simulink model "PMSM_simplified"  (R2023a)
settings: Solver=VariableStepAuto  StartTime=0.0  StopTime=1  RelTol=1e-3
libraries: spsVoltageMeasurementLib x3, spsGroundLib x1, spsPermanentMagnetSynchronousMachineLib x1, spsThreePhaseProgrammableVoltageSourceLib x1, sps_lib x1
settings Model: Creator=siddh  LastModifiedBy=siddh

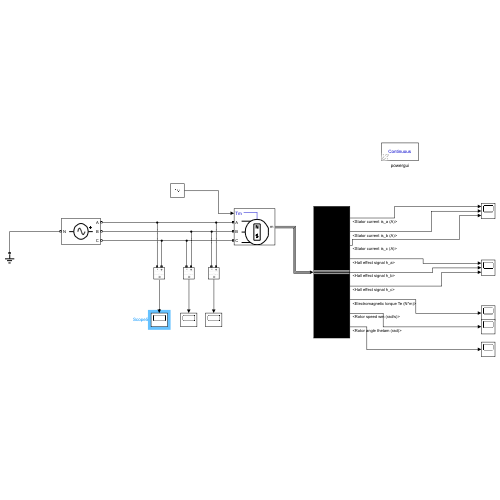
[thumbnail: Simulink's stored preview of the top-level diagram]
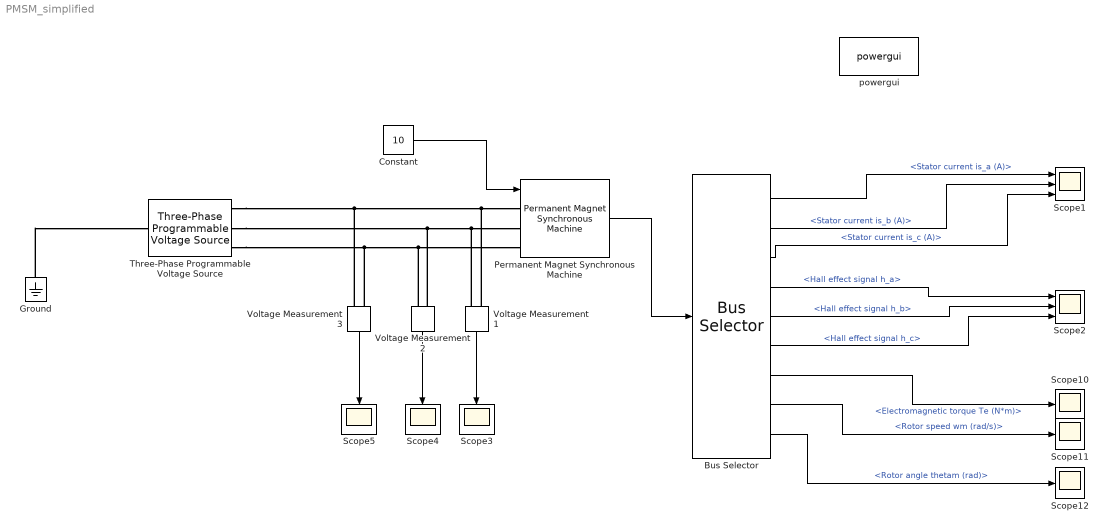
== system PMSM_simplified ==
  Bus Selector : BusSelector  OutputSignals=Stator current is_a (A),Stator current is_b (A),Stator current is_c (A),Hall effect signal h_a,Hall effect signal h_b,Hall effect signal h_c,Electromagnetic torque Te (N*m),Rotor speed wm (rad/s),Rotor angle thetam (rad)
  Constant : Constant  Value=10
  Ground : spsGroundLib/Ground  LConnTagsString=a
  Permanent Magnet Synchronous Machine : spsPermanentMagnetSynchronousMachineLib/Permanent Magnet Synchronous Machine  NbPhases=3  FluxDistribution=Sinusoidal  RotorType=Round  MechanicalLoad=Torque Tm  PresetModel=No  ShowDetailedParameters=on  MeasurementBus=off  Resistance=18.7  Inductance=8.5e-3  dqInductances=[8.5e-3,8.5e-3]  La=0.02682  MachineConstant=Flux linkage established by magnets (V.s)  Flux=0.1716  VoltageCst=62.2496  TorqueCst=0.5148  Flat=120  Mechanical=[2.26e-05 1.349e-05 2 0]  PolePairs=2  InitialConditions=[0,0, 0,0]  InitialConditions5ph=[0 0 0 0 0 0]  RefAngle=90 degrees behind phase A axis (modified Park)  IterativeDiscreteModel=Trapezoidal non iterative  TsBlock=-1  TsPowergui=0
  Scope1 : Scope  NumInputPorts=3
  Scope{3..5,10..12} (6 alike) : Scope
  Scope2 : Scope  NumInputPorts=3
  Three-Phase Programmable Voltage Source : spsThreePhaseProgrammableVoltageSourceLib/Three-Phase Programmable Voltage Source  PositiveSequence="[100  0 50]"  VariationEntity=None  VariationType=Table of time-amplitude pairs  VariationTypeAlt=Step  VariationStep=0.5  VariationRate=10  VariationMagnitude=0.3  VariationFrequency=2  VariationTiming=[1 2]  VariationPhaseA=off  Amplitudes=[1 0.8 1.2 1.0]  TimeValues=[0 0.1 0.15 0.2]  HarmonicGeneration=off  HarmonicA=[3 0.2 -25 0]  HarmonicB=[2 0.15 35 2]  Timing="[0.05  3]"  BusType=swing  Pref=0  Qref=0  Qmin=-inf  Qmax=inf
  Voltage Measurement1 : spsVoltageMeasurementLib/Voltage Measurement  PhasorSimulation=off  OutputType=Complex  PSBequivalent=0
  Voltage Measurement2 : spsVoltageMeasurementLib/Voltage Measurement  PhasorSimulation=off  OutputType=Complex  PSBequivalent=0
  Voltage Measurement3 : spsVoltageMeasurementLib/Voltage Measurement  PhasorSimulation=off  OutputType=Complex  PSBequivalent=0
  powergui : sps_lib/powergui  Priority=1  SimulationMode=Continuous  SampleTime=50e-6  frequency=60  Iterations=50  frequencyindice=0  Pbase=100e6  ErrMax=1e-4  UnitsV=kV  UnitsW=MW  buscounter=0  FunctionMessages=off  echomessages=off  EnableUseOfTLC=off  CurrentSourceSwitches=off  DisableSnubberDevices=off  DisableRonSwitches=off  DisableVfSwitches=off  DisplayEquations=off  AutomaticDiscreteSolvers=off  SolverType=Tustin/Backward Euler (TBE)  Interpol=off  ExternalGateDelay=off  methode=off  Ts=100  x0status=blocks  SPID=on  SwTol=0  HookPort=off  NonlinearTolerance=1e-4  nMaxIteration=100  ContinueOnMaxIteration=off  RestoreLinks=warning  ResistiveCurrentMeasurement=off  Frange=[0:2:500]  Ylog=off  Xlog=on  ShowGrid=off  save=off  variable=ZData  structure=0  ZoomFFT=off  StartTime=0.0  cycles=1  DisplayStyle=1  fundamental=60  FreqAxis=off  MaxFrequency=1000  frequencyindicesteady=1  RmsSteady=1  display=off
  wires:
  Bus Selector/6 -> Scope2/3  "<Hall effect signal h_c>"
  Bus Selector/7 -> Scope10/1  "<Electromagnetic torque Te (N*m)>"
  Constant/1 -> Permanent Magnet Synchronous Machine/1
  Permanent Magnet Synchronous Machine/1 -> Bus Selector/1
  Bus Selector/2 -> Scope1/2  "<Stator current is_b (A)>"
  Bus Selector/8 -> Scope11/1  "<Rotor speed wm (rad/s)>"
  Bus Selector/1 -> Scope1/1  "<Stator current is_a (A)>"
  Bus Selector/3 -> Scope1/3  "<Stator current is_c (A)>"
  Bus Selector/9 -> Scope12/1  "<Rotor angle thetam (rad)>"
  Bus Selector/4 -> Scope2/1  "<Hall effect signal h_a>"
  Bus Selector/5 -> Scope2/2  "<Hall effect signal h_b>"
  Voltage Measurement1/1 -> Scope3/1
  Voltage Measurement2/1 -> Scope4/1
  Voltage Measurement3/1 -> Scope5/1
  connections:
  Three-Phase Programmable Voltage Source/RConn1 -- Voltage Measurement3/LConn2 -- Voltage Measurement1/LConn1 -- Permanent Magnet Synchronous Machine/LConn1
  Three-Phase Programmable Voltage Source/RConn2 -- Voltage Measurement1/LConn2 -- Permanent Magnet Synchronous Machine/LConn2 -- Voltage Measurement2/LConn1
  Three-Phase Programmable Voltage Source/RConn3 -- Voltage Measurement3/LConn1 -- Voltage Measurement2/LConn2 -- Permanent Magnet Synchronous Machine/LConn3
  Ground/LConn1 -- Three-Phase Programmable Voltage Source/LConn1
